simulink model "bike_model_2states_smithSteering"  (R2018b)
settings: Solver=VariableStepAuto  StartTime=0.0  StopTime=sim_time  FixedStep=Ts/10  MaxStep=Ts/10
values from neighbouring files (symbols this model uses):
  A_bike = [0 g/h_real ; 1 0]    [configuration.m]
  B_bike = [1 ; 0]    [configuration.m]
  b_compFilter = 1.095    [configuration.m]    (also in configuration_pidTuning.m)
  b_real = 1.095    [configuration.m]    (also in configuration_pidTuning.m)
  C1_bike = a_real/(b_real*h_real)    (= 0.392543973584)    [configuration.m]
  C2_bike = 1/(b_real*h_real)    (= 1.15454109878)    [configuration.m]
  C_ini = [C1_bike*input_velocity C2_bike*input_velocity^2]    [configuration.m]
  complementary = 0.985    [configuration.m]    (also in configuration_pidTuning.m)
  D = zeros(3,1)    [configuration_pidTuning.m]
  D_steering_position = 0.0    (= 0)    [configuration.m]
  Dead_Band = [0.055, -0.055, 0.005]    [configuration.m]    (also in configuration_pidTuning.m)
  delay = 0.045    [configuration.m]    (also in configuration_pidTuning.m)
  delay_tf_steering = 0    [configuration.m]
  den_tf_steering = [1 245.9 0]    [configuration.m]
  den_tf_steering_dis = [den_tf_steering_dis 0] - [0 den_tf_steering_dis]    [configuration.m]
  direct_control = 1    [configuration.m]    (also in configuration_pidTuning.m)
  f_filter_phidot = 20    [configuration.m]
  filter_model = 1    [configuration.m]    (also in configuration_pidTuning.m)
  forward_motor_dynamics = 0    [configuration.m]    (also in configuration_pidTuning.m)
  forward_speed_offset = 0    [configuration.m]
  g = 9.81    [configuration.m]    (also in configuration_pidTuning.m)
  I_direct = 0.000227125326188444    (= 0.000227125326188)    [configuration.m]    (also in configuration_pidTuning.m)
  I_lat = 0.000115580509653549    (= 0.000115580509654)    [configuration.m]    (also in configuration_pidTuning.m)
  I_steering_position = 1    [configuration.m]    (also in simulate_bike.m = 30)
  IMU_height_model = 0.45    [configuration.m]    (also in configuration_pidTuning.m)
  IMU_height_real = 0.45    [configuration.m]    (also in configuration_pidTuning.m)
  initial_states = [deg2rad(-2) deg2rad(0) deg2rad(0)]    [configuration.m]    (also in configuration_pidTuning.m)
  input_velocity = 4    [configuration.m]    (also in configuration_pidTuning.m = 3)
  lambda_compFilter = deg2rad(70)    [configuration.m]    (also in configuration_pidTuning.m)
  lambda_real = deg2rad(70)    [configuration.m]    (also in configuration_pidTuning.m)
  lat_control = 0    [configuration.m]    (also in configuration_pidTuning.m = 1)
  look_ahead = 0    [configuration.m]    (also in configuration_pidTuning.m)
  lqr_gains = zeros(length(velocity_lqr),1+size(A_bike,1))    [lqr_design.m]
  max_handlebar = 40*(pi/180)    (= 0.698131700798)    [configuration.m]    (also in configuration_pidTuning.m)
  max_roll = pi/2    (= 1.57079632679)    [configuration.m]    (also in configuration_pidTuning.m)
  max_steering_motor_acc = inf    [configuration.m]    (also in configuration_pidTuning.m)
  max_steering_motor_speed = 0.9    [configuration.m]    (also in configuration_pidTuning.m = 7.5)
  min_handlebar = -max_handlebar    (= -0.698131700798)    [configuration.m]    (also in configuration_pidTuning.m)
  min_roll = - max_roll    (= -1.57079632679)    [configuration.m]    (also in configuration_pidTuning.m)
  min_steering_motor_acc = -inf    [configuration.m]    (also in configuration_pidTuning.m)
  min_steering_motor_speed = -0.9    [configuration.m]    (also in configuration_pidTuning.m = -7.5)
  noise = 0    [configuration.m]    (also in configuration_pidTuning.m)
  noise_acc = 2.4869e-05    [configuration.m]    (also in configuration_pidTuning.m)
  noise_encoder = 1e-7    (= 1e-07)    [configuration.m]    (also in configuration_pidTuning.m)
  noise_gyro = 0.005    [configuration.m]    (also in configuration_pidTuning.m = 0.0022)
  noise_hall = 0.0031    [configuration.m]    (also in configuration_pidTuning.m)
  noise_pos_meas = 0    [configuration.m]    (also in configuration_pidTuning.m = 0.51)
  num_tf_steering = [253.4]    [configuration.m]
  num_tf_steering_dis = [num_tf_steering_dis 0]    [configuration.m]
  offset_acc = 0.0*g    (= 0)    [configuration.m]
  offset_encoder = deg2rad(1)    [configuration.m]
  offset_gyro = deg2rad(0)    [configuration.m]
  offset_hall = 0.0    (= 0)    [configuration.m]
  offset_pos_x = 0    [configuration.m]
  offset_pos_y = 0    [configuration.m]
  P_direct = 0.0712859744206787    (= 0.0712859744207)    [configuration.m]    (also in configuration_pidTuning.m)
  P_lat = 0.0465435246389258    (= 0.0465435246389)    [configuration.m]    (also in configuration_pidTuning.m)
  P_steering_position = 10    [configuration.m]    (also in simulate_bike.m = 30)
  parameters_compFilter = [g h_compFilter b_compFilter a_compFilter lambda_compFilter c_compFilter]    [configuration.m]    (also in configuration_pidTuning.m)
  roll_rate_coef = 0.9    [configuration.m]    (also in configuration_pidTuning.m)
  sensor_offset = 0    [configuration.m]
  smith_steering = 0    [configuration.m]
  steering_angle_correction = deg2rad(0)    [configuration.m]
  steering_motor_limitations = 0    [configuration.m]    (also in configuration_pidTuning.m = 1)
  sys_con = ss(A_lqr,B_lqr,C_lqr,D_lqr)    [lqr_design.m]
  time_offset_acc = 7    [configuration.m]
  time_offset_encoder = 10    [configuration.m]
  time_offset_gyro = 7    [configuration.m]
  time_offset_hall = 7    [configuration.m]
  time_offset_pos_x = 7    [configuration.m]
  time_offset_pos_y = 7    [configuration.m]
  Ts = 0.01    [configuration.m]    (also in configuration_pidTuning.m = 0.04)
  Ts_IMU = 0.01    [configuration.m]    (also in configuration_pidTuning.m = 0.04)
  velocity_lqr = [input_velocity - 0.1 , input_velocity , input_velocity + 0.1]    [lqr_design.m]
undefined symbols (not defined in the file or in its folder): A, B, cumulative_dist_along_path, curvature, den_filter_phidot, initial_x, initial_y, num_filter_phidot, path_x, path_y
libraries: simulink x17, simulink_extras x3, dspsigops x2
(part 2 of 3)

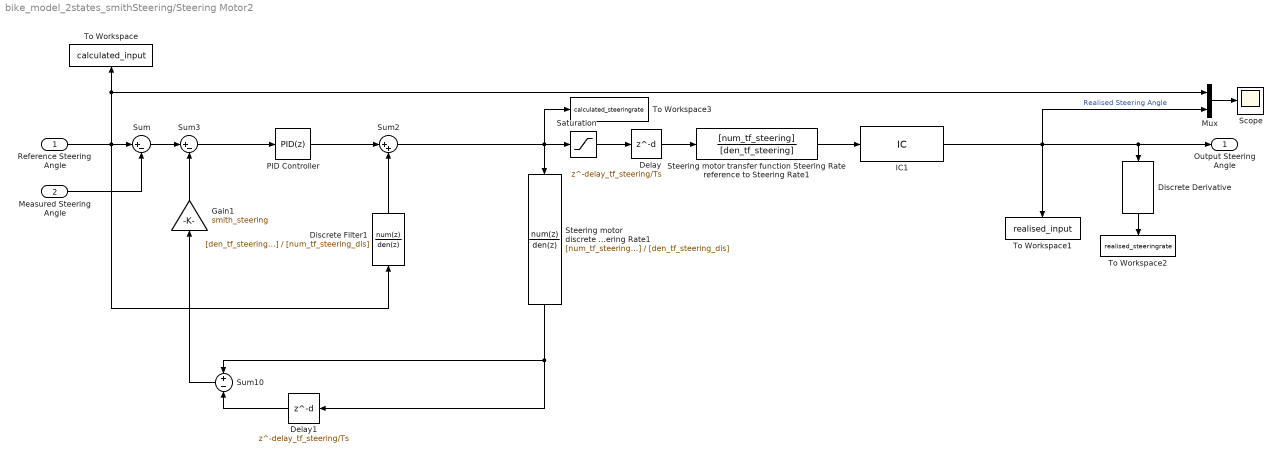
== system bike_model_2states_smithSteering/Steering Motor2 ==
  Reference Steering Angle : Inport
  Measured Steering Angle : Inport  Port=2
  Delay : Delay  DelayLength=delay_tf_steering/Ts  SampleTime=Ts
  Delay1 : Delay  DelayLength=delay_tf_steering/Ts  SampleTime=Ts
  Discrete Derivative : simulink/Discrete/Discrete Derivative  gainval=1.0  ICPrevScaledInput=0.0  OutMin=[]  OutMax=[]  OutDataType=fixdt(1, 16)  OutScaling=2^-10  DoSatur=off
  Discrete Filter1 : DiscreteFilter  Numerator=[den_tf_steering_dis]  Denominator=[num_tf_steering_dis]
  Gain1 : Gain  Gain=smith_steering
  IC1 : InitialCondition  Value=initial_states(2)
  Mux : Mux  Inputs=2
  PID Controller : simulink/Continuous/PID Controller  Controller=PID  Form=Parallel  TimeDomain=Discrete-time  SampleTime=Ts  IntegratorMethod=Forward Euler  FilterMethod=Forward Euler  ControllerParametersSource=internal  P=P_steering_position  I=I_steering_position  D=D_steering_position  UseFilter=off  N=1  TunerSelectOption=Transfer Function Based (PID Tuner App)  InitialConditionSource=internal  InitialConditionForIntegrator=0  InitialConditionForFilter=0  DifferentiatorICPrevScaledInput=0  ExternalReset=none  TrackingMode=off  Kt=1  LimitOutput=off  UpperSaturationLimit=inf  LowerSaturationLimit=-inf  LinearizeAsGain=on  AntiWindupMode=none  Kb=1  POutMin=[]  POutMax=[]  IOutMin=[]  IOutMax=[]  DOutMin=[]  DOutMax=[]  NOutMin=[]  NOutMax=[]  SumOutMin=[]  SumOutMax=[]  SaturationOutMin=[]  SaturationOutMax=[]  PParamMin=[]  PParamMax=[]  IParamMin=[]  IParamMax=[]  DParamMin=[]  DParamMax=[]  NParamMin=[]  NParamMax=[]  KbParamMin=[]  KbParamMax=[]  KtParamMin=[]  KtParamMax=[]  KbOutMin=[]  KbOutMax=[]  KtOutMin=[]  KtOutMax=[]  IntegratorOutMin=[]  IntegratorOutMax=[]  FilterOutMin=[]  FilterOutMax=[]  SumI1OutMin=[]  SumI1OutMax=[]  SumI2OutMin=[]  SumI2OutMax=[]  SumI3OutMin=[]  SumI3OutMax=[]  SumI4OutMin=[]  SumI4OutMax=[]  SumDOutMin=[]  SumDOutMax=[]  DifferentiatorOutMin=[]  DifferentiatorOutMax=[]  FilterDiffOutCoefMin=[]  FilterDiffOutCoefMax=[]  ReciprocalOutMin=[]  ReciprocalOutMax=[]  SumDenOutMin=[]  SumDenOutMax=[]  SumNumOutMin=[]  SumNumOutMax=[]  DivideOutMin=[]  DivideOutMax=[]  IntegratorContinuousStateAttributes=''  IntegratorStateMustResolveToSignalObject=off  IntegratorRTWStateStorageClass=Auto  FilterContinuousStateAttributes=''  FilterStateMustResolveToSignalObject=off  FilterRTWStateStorageClass=Auto  ParallelPVariant=InternalParameters  IdealPVariant=Disabled  IVariant=InternalParameters  DVariant=InternalParameters  IntegratorVariant=Discrete  SatVariant=Disabled  AWVariant=Passthrough  PCopyVariant=Disabled  TRVariant=Disabled  FdbkBlocksVariant=Forward  IdealPFdbkVariant=Disabled  SatFdbkVariant=Disabled  DerivativeFilterVariant=Differentiator  NVariant=Passthrough  NCopyVariant=Disabled_SignalSpec  FilterICVariant=InternalICsDifferentiator  IntegratorICVariant=InternalICs  ExternalResetVariant=Disabled  TRSumVariant=Passthrough  SumFdbkVariant=Disabled  SumVariant=Sum_PID
  Saturation : Saturate  UpperLimit=max_steering_motor_speed  LowerLimit=min_steering_motor_speed
  Scope : Scope
  Steering motor discrete transfer function Steering Rate reference to Steering Rate1 : DiscreteTransferFcn  Numerator=[num_tf_steering_dis]  Denominator=[den_tf_steering_dis]  SampleTime=Ts
  Steering motor transfer function Steering Rate reference to Steering Rate1 : TransferFcn  Numerator=[num_tf_steering]  Denominator=[den_tf_steering]
  Sum : Sum  Inputs=|+-
  Sum10 : Sum  Inputs=+-
  Sum2 : Sum  Inputs=|++
  Sum3 : Sum  Inputs=|+-
  To Workspace : ToWorkspace  VariableName=calculated_input  SaveFormat=Timeseries  SampleTime=Ts
  To Workspace1 : ToWorkspace  VariableName=realised_input  SaveFormat=Timeseries  SampleTime=-1
  To Workspace2 : ToWorkspace  VariableName=realised_steeringrate  SaveFormat=Timeseries  SampleTime=-1
  To Workspace3 : ToWorkspace  VariableName=calculated_steeringrate  SaveFormat=Timeseries  SampleTime=-1
  Output Steering Angle : Outport
  wires:
  Mux/1 -> Scope/1
  Delay/1 -> Steering motor transfer function Steering Rate reference to Steering Rate1/1
  PID Controller/1 -> Sum2/1
  Reference Steering Angle/1 -> Discrete Filter1/1, Sum/1, Mux/1, To Workspace/1
  Sum2/1 -> To Workspace3/1, Steering motor discrete transfer function Steering Rate reference to Steering Rate1/1, Saturation/1
  Measured Steering Angle/1 -> Sum/2
  Sum/1 -> Sum3/1
  Delay1/1 -> Sum10/2
  Steering motor discrete transfer function Steering Rate reference to Steering Rate1/1 -> Delay1/1, Sum10/1
  Sum10/1 -> Gain1/1
  Steering motor transfer function Steering Rate reference to Steering Rate1/1 -> IC1/1
  IC1/1 -> To Workspace1/1, Discrete Derivative/1, Output Steering Angle/1, Mux/2  "Realised Steering Angle"
  Discrete Filter1/1 -> Sum2/2
  Sum3/1 -> PID Controller/1
  Saturation/1 -> Delay/1
  Discrete Derivative/1 -> To Workspace2/1
  Gain1/1 -> Sum3/2

== system bike_model_2states_smithSteering/Balance Controller/LQR Controller ==
  note: Input = steering angular velocity
  Velocity : Inport
  State Error : Inport  Port=2
  1-D Lookup Table : Lookup_n-D  NumberOfTableDimensions=1  BreakpointsForDimension1=velocity_lqr  BreakpointsForDimension2=velocity_lqr  BreakpointsForDimension3=velocity_lqr  BreakpointsForDimension4=velocity_lqr  Table=lqr_gains(:,1)  InternalRulePriority=Speed  RndMeth=Simplest  InputSameDT=on
  1-D Lookup Table1 : Lookup_n-D  NumberOfTableDimensions=1  BreakpointsForDimension1=velocity_lqr  BreakpointsForDimension2=velocity_lqr  BreakpointsForDimension3=velocity_lqr  BreakpointsForDimension4=velocity_lqr  Table=lqr_gains(:,2)  InternalRulePriority=Speed  RndMeth=Simplest  InputSameDT=on
  Display1 : Display
  Mux : Mux  Inputs=2
  Product : Product  Multiplication=Matrix(*)
  Scope : Scope
  Transpose : Math  Operator=transpose  SaturateOnIntegerOverflow=on
  Zero-Order Hold : ZeroOrderHold  SampleTime=Ts
  Zero-Order Hold1 : ZeroOrderHold  SampleTime=Ts
  Calculated Input : Outport
  wires:
  1-D Lookup Table/1 -> Mux/1  "K1"
  1-D Lookup Table1/1 -> Mux/2  "K2"
  State Error/1 -> Zero-Order Hold1/1
  Product/1 -> Zero-Order Hold/1
  Velocity/1 -> 1-D Lookup Table1/1, 1-D Lookup Table/1
  Mux/1 -> Product/2, Display1/1
  Transpose/1 -> Product/1
  Zero-Order Hold/1 -> Calculated Input/1
  Zero-Order Hold1/1 -> Scope/1, Transpose/1

== system bike_model_2states_smithSteering/Balance Controller/Reference States Generator ==
  Velocity : Inport
  Steering Angle : Inport  Port=2
  Angles Error : Inport  Port=3
  Constant1 : Constant  Value=A_bike
  Constant2 : Constant  Value=0
  Constant3 : Constant  Value=B_bike
  Gain : Gain  Gain=C2_bike
  Gain1 : Gain  Gain=C1_bike
  Matrix Concatenate : Concatenate  Mode=Multidimensional array
  Mux1 : Mux  Inputs=2
  Mux2 : Mux  Inputs=2
  Product{1..4} (4 alike) : Product  SCDEnableBlockLinearizationSpecification=on  Multiplication=Matrix(*)
  Product5 : Product  SCDEnableBlockLinearizationSpecification=on  Inputs=/  Multiplication=Matrix(*)
  Reshape : Reshape  OutputDimensionality=Row vector (2-D)
  Square1 : Math  Operator=square  SaturateOnIntegerOverflow=on
  Sum : Sum  Inputs=-+
  State Error : Outport
  wires:
  Velocity/1 -> Square1/1, Gain1/1
  Square1/1 -> Gain/1
  Reshape/1 -> Product4/1, Matrix Concatenate/1, Product3/1  "C"
  Mux2/1 -> Reshape/1
  Constant1/1 -> Product3/2  "A"
  Product3/1 -> Matrix Concatenate/2  "CA"
  Matrix Concatenate/1 -> Product5/1  "[C ; CA]"
  Angles Error/1 -> Sum/2
  Product2/1 -> Sum/1
  Steering Angle/1 -> Product2/2
  Mux1/1 -> Product2/1  "[0 ; CB]"
  Constant2/1 -> Mux1/1
  Product4/1 -> Mux1/2
  Constant3/1 -> Product4/2  "B"
  Sum/1 -> Product1/2
  Product1/1 -> State Error/1  "CA"
  Product5/1 -> Product1/1  "CA"
  Gain1/1 -> Mux2/1
  Gain/1 -> Mux2/2

== system bike_model_2states_smithSteering/Balance Controller1/LQR Controller ==
  Velocity : Inport
  State Error : Inport  Port=2
  1-D Lookup Table : Lookup_n-D  NumberOfTableDimensions=1  BreakpointsForDimension1=velocity_lqr  BreakpointsForDimension2=velocity_lqr  BreakpointsForDimension3=velocity_lqr  BreakpointsForDimension4=velocity_lqr  Table=lqr_gains(:,2)  InternalRulePriority=Speed  RndMeth=Simplest  InputSameDT=on
  1-D Lookup Table1 : Lookup_n-D  NumberOfTableDimensions=1  BreakpointsForDimension1=velocity_lqr  BreakpointsForDimension2=velocity_lqr  BreakpointsForDimension3=velocity_lqr  BreakpointsForDimension4=velocity_lqr  Table=lqr_gains(:,3)  InternalRulePriority=Speed  RndMeth=Simplest  InputSameDT=on
  Display1 : Display
  Mux : Mux  Inputs=2
  Product : Product  Multiplication=Matrix(*)
  Transpose : Math  Operator=transpose  SaturateOnIntegerOverflow=on
  Zero-Order Hold : ZeroOrderHold  SampleTime=Ts
  Calculated Input : Outport
  wires:
  1-D Lookup Table/1 -> Mux/1  "K1"
  1-D Lookup Table1/1 -> Mux/2  "K2"
  Product/1 -> Zero-Order Hold/1
  Velocity/1 -> 1-D Lookup Table1/1, 1-D Lookup Table/1
  Mux/1 -> Product/2, Display1/1
  Transpose/1 -> Product/1
  Zero-Order Hold/1 -> Calculated Input/1
  State Error/1 -> Transpose/1

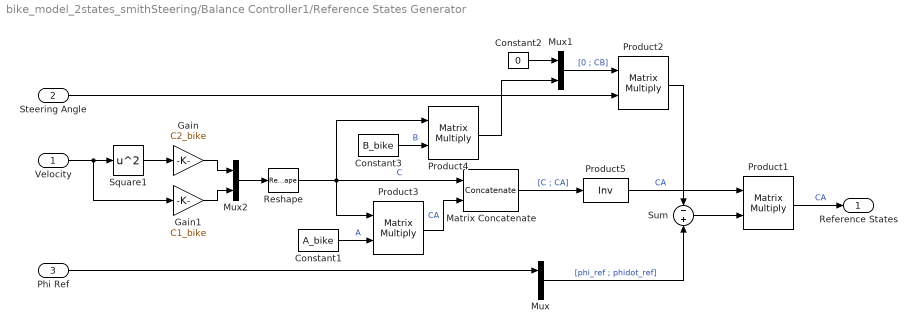
== system bike_model_2states_smithSteering/Balance Controller1/Reference States Generator ==
  Velocity : Inport
  Steering Angle : Inport  Port=2
  Phi Ref : Inport  Port=3
  Constant1 : Constant  Value=A_bike
  Constant2 : Constant  Value=0
  Constant3 : Constant  Value=B_bike
  Gain : Gain  Gain=C2_bike
  Gain1 : Gain  Gain=C1_bike
  Matrix Concatenate : Concatenate  Mode=Multidimensional array
  Mux : Mux  Inputs=2
  Mux1 : Mux  Inputs=2
  Mux2 : Mux  Inputs=2
  Product{1..4} (4 alike) : Product  SCDEnableBlockLinearizationSpecification=on  Multiplication=Matrix(*)
  Product5 : Product  SCDEnableBlockLinearizationSpecification=on  Inputs=/  Multiplication=Matrix(*)
  Reshape : Reshape  OutputDimensionality=Row vector (2-D)
  Square1 : Math  Operator=square  SaturateOnIntegerOverflow=on
  Sum : Sum  Inputs=-+
  Reference States : Outport
  wires:
  Velocity/1 -> Gain1/1, Square1/1
  Gain1/1 -> Mux2/2
  Gain/1 -> Mux2/1
  Square1/1 -> Gain/1
  Reshape/1 -> Product4/1, Matrix Concatenate/1, Product3/1  "C"
  Mux2/1 -> Reshape/1
  Constant1/1 -> Product3/2  "A"
  Product3/1 -> Matrix Concatenate/2  "CA"
  Matrix Concatenate/1 -> Product5/1  "[C ; CA]"
  Mux/1 -> Sum/2  "[phi_ref ; phidot_ref]"
  Phi Ref/1 -> Mux/1
  Product2/1 -> Sum/1
  Steering Angle/1 -> Product2/2
  Mux1/1 -> Product2/1  "[0 ; CB]"
  Constant2/1 -> Mux1/1
  Product4/1 -> Mux1/2
  Constant3/1 -> Product4/2  "B"
  Sum/1 -> Product1/2
  Product1/1 -> Reference States/1  "CA"
  Product5/1 -> Product1/1  "CA"

== system bike_model_2states_smithSteering/Complementary filter/Complementary Filter ==
  Roll Angle Estimation due to Accelerometer : Inport
  Roll Rate due to Gyroscope : Inport  Port=2
  Delay : Delay  DelayLength=1  InitialCondition=initial_states(1)
  Gain2 : Gain  Gain=complementary
  Gain3 : Gain  Gain=1-complementary
  Gain4 : Gain  Gain=Ts_IMU
  Sum3 : Sum  Inputs=|++
  Sum4 : Sum  Inputs=++|
  Roll Angle Estimation : Outport
  wires:
  Roll Angle Estimation due to Accelerometer/1 -> Gain3/1  "Roll_acc"
  Sum3/1 -> Gain2/1
  Roll Rate due to Gyroscope/1 -> Gain4/1
  Delay/1 -> Sum3/2
  Gain4/1 -> Sum3/1
  Gain2/1 -> Sum4/2
  Gain3/1 -> Sum4/1
  Sum4/1 -> Delay/1, Roll Angle Estimation/1

== system bike_model_2states_smithSteering/Complementary filter/Roll Angle Estimation of Accelerometer ==
  Accelerations : Inport
  Measured Steering Angle : Inport  Port=2
  Measured Velocity : Inport  Port=3
  Steering Rate : Inport  Port=4
  Roll Rate : Inport  Port=5
  Measured Roll Angle : Inport  Port=6
  Atan2 : Trigonometry  Operator=atan2
  Centripetal Acceleration Compensator : Subsystem
  Cos : Trigonometry  Operator=cos
  Demux : Demux  Outputs=3
  Lateral Acceleration Compensator : Subsystem
  Multiply : Product
  Multiply1 : Product
  Sin : Trigonometry
  Sum1 : Sum  Inputs=-+
  Sum6 : Sum  Inputs=+-+
  Roll Angle Estimation of Accelerometer : Outport
  wires:
  Sum1/1 -> Atan2/2
  Lateral Acceleration Compensator/1(Estimated Lateral Accelerattion due to Roll) -> Sum6/1
  Atan2/1 -> Roll Angle Estimation of Accelerometer/1  "Roll_acc"
  Roll Rate/1 -> Lateral Acceleration Compensator/4(Roll Rate)
  Accelerations/1 -> Demux/1
  Measured Velocity/1 -> Lateral Acceleration Compensator/1(Measured Velocity), Centripetal Acceleration Compensator/2(Velocity)
  Measured Steering Angle/1 -> Lateral Acceleration Compensator/3(Steering Angle), Centripetal Acceleration Compensator/1(Steering Angle)
  Centripetal Acceleration Compensator/1(Estimated Centripetal Acceleration) -> Multiply/2, Multiply1/1
  Measured Roll Angle/1 -> Lateral Acceleration Compensator/2(Roll Angle), Sin/1, Cos/1
  Cos/1 -> Multiply1/2
  Sin/1 -> Multiply/1
  Multiply1/1 -> Sum6/2
  Demux/3 -> Sum1/2
  Multiply/1 -> Sum1/1
  Steering Rate/1 -> Lateral Acceleration Compensator/5(Steering Rate)
  Sum6/1 -> Atan2/1
  Demux/2 -> Sum6/3

== system bike_model_2states_smithSteering/Complementary filter2/Complementary Filter ==
  Roll Angle Estimation due to Accelerometer : Inport
  Roll Rate due to Gyroscope : Inport  Port=2
  Delay : Delay  DelayLength=1  InitialCondition=initial_states(1)
  Gain2 : Gain  Gain=complementary
  Gain3 : Gain  Gain=1-complementary
  Gain4 : Gain  Gain=Ts_IMU
  Sum3 : Sum  Inputs=|++
  Sum4 : Sum  Inputs=++|
  Roll Angle Estimation : Outport
  wires:
  Roll Angle Estimation due to Accelerometer/1 -> Gain3/1  "Roll_acc"
  Sum3/1 -> Gain2/1
  Roll Rate due to Gyroscope/1 -> Gain4/1
  Delay/1 -> Sum3/2
  Gain4/1 -> Sum3/1
  Gain2/1 -> Sum4/2
  Gain3/1 -> Sum4/1
  Sum4/1 -> Delay/1, Roll Angle Estimation/1

== system bike_model_2states_smithSteering/Complementary filter2/Roll Angle Estimation of Accelerometer ==
  Accelerations : Inport
  Roll Rate : Inport  Port=2
  Measured Steering Angle : Inport  Port=3
  Measured Velocity : Inport  Port=4
  Measured Roll Angle : Inport  Port=5
  Steering Rate : Inport  Port=6
  Atan2 : Trigonometry  Operator=atan2
  Centripetal Acceleration Compensator : Subsystem
  Cos : Trigonometry  Operator=cos
  Demux : Demux  Outputs=3
  Lateral Acceleration Compensator : Subsystem
  Multiply : Product
  Multiply1 : Product
  Saturation -90°/90° : Saturate  UpperLimit=max_roll  LowerLimit=min_roll
  Sin : Trigonometry
  Sum1 : Sum  Inputs=-+
  Sum6 : Sum  Inputs=+-+
  Roll Angle Estimation of Accelerometer : Outport
  wires:
  Sum1/1 -> Atan2/2
  Lateral Acceleration Compensator/1(Estimated Lateral Accelerattion due to Roll) -> Sum6/1
  Atan2/1 -> Saturation -90°/90°/1  "Roll_acc"
  Roll Rate/1 -> Lateral Acceleration Compensator/4(Roll Rate)
  Accelerations/1 -> Demux/1
  Measured Velocity/1 -> Lateral Acceleration Compensator/1(Measured Velocity), Centripetal Acceleration Compensator/2(Velocity)
  Measured Steering Angle/1 -> Lateral Acceleration Compensator/3(Steering Angle)
  Centripetal Acceleration Compensator/1(Estimated Centripetal Acceleration) -> Multiply/2, Multiply1/1
  Measured Roll Angle/1 -> Lateral Acceleration Compensator/2(Roll Angle), Sin/1, Cos/1
  Cos/1 -> Multiply1/2
  Sin/1 -> Multiply/1
  Multiply1/1 -> Sum6/2
  Demux/3 -> Sum1/2
  Multiply/1 -> Sum1/1
  Steering Rate/1 -> Lateral Acceleration Compensator/5(Steering Rate)
  Sum6/1 -> Atan2/1
  Lateral Acceleration Compensator/2(Steering Angle (temporary output)) -> Centripetal Acceleration Compensator/1(Steering Angle)
  Demux/2 -> Sum6/3
  Saturation -90°/90°/1 -> Roll Angle Estimation of Accelerometer/1

== system bike_model_2states_smithSteering/Global Angles and Coordinates Calculator - Velocity/Measured Bike Angles to Global Angles ==
  note: Verification of the equivalence of the calculus for Beta estimation
  Velocity : Inport
  Measured Steering Angle : Inport  Port=2
  Gain : Gain  Gain=1/b_compFilter
  Integrator : Integrator
  MATLAB Function : MATLAB Function  TreatAsAtomicUnit=on
  Multiply : Product
  Parameters : Constant  Value=parameters_compFilter
  Scope : Scope  NumInputPorts=2
  Tan : Trigonometry  Operator=tan
  Psi : Outport
  Beta : Outport  Port=2
  wires:
  Integrator/1 -> Psi/1
  MATLAB Function/1(psi_d) -> Scope/1, Integrator/1
  Measured Steering Angle/1 -> Tan/1, MATLAB Function/3(delta)
  Parameters/1 -> MATLAB Function/2(parameters_model)
  Velocity/1 -> Multiply/1, MATLAB Function/1(v)
  MATLAB Function/2(beta) -> Beta/1
  Tan/1 -> Multiply/2
  Multiply/1 -> Gain/1
  Gain/1 -> Scope/2

== system bike_model_2states_smithSteering/Global Angles and Coordinates Calculator - Velocity/Measured Global Angles to Global Coordinates ==
  Velocity : Inport
  Psi : Inport  Port=2
  Beta : Inport  Port=3
  MATLAB Function1 : MATLAB Function  TreatAsAtomicUnit=on
  Mux1 : Mux  Inputs=2
  "Velocity (Xdot, Ydot)" : Outport
  wires:
  MATLAB Function1/2(Ydot) -> Mux1/2  "Ydot"
  MATLAB Function1/1(Xdot) -> Mux1/1  "Xdot"
  Psi/1 -> MATLAB Function1/2(psi)
  Beta/1 -> MATLAB Function1/3(beta)
  Velocity/1 -> MATLAB Function1/1(v)
  Mux1/1 -> "Velocity (Xdot, Ydot)"/1

== system bike_model_2states_smithSteering/IMU/IMU Accelerometer ==
  Lateral Acceleration of the IMU due to Roll : Inport
  Centripetal Acceleration due to Path Curvature : Inport  Port=2
  True Velocity : Inport  Port=3
  True Roll Angle : Inport  Port=4
  Cos : Trigonometry  Operator=cos
  Derivative : Derivative  CoefficientInTFapproximation=-1
  Gain1 : Gain  Gain=g
  Gain2 : Gain  Gain=g
  Multiply : Product
  Multiply1 : Product
  Mux : Mux  Inputs=3
  Sin : Trigonometry
  Sum1 : Sum  Inputs=-+
  Sum6 : Sum  Inputs=-++
  Accelerations : Outport
  wires:
  Multiply/1 -> Sum6/2
  Gain1/1 -> Sum6/3  "acc_y"
  Sin/1 -> Multiply1/2, Gain1/1
  Derivative/1 -> Mux/1  "acc_x"
  Cos/1 -> Multiply/2, Gain2/1
  Gain2/1 -> Sum1/2  "acc_z"
  True Roll Angle/1 -> Sin/1, Cos/1
  True Velocity/1 -> Derivative/1
  Centripetal Acceleration due to Path Curvature/1 -> Multiply1/1, Multiply/1
  Multiply1/1 -> Sum1/1
  Sum1/1 -> Mux/3
  Mux/1 -> Accelerations/1
  Sum6/1 -> Mux/2
  Lateral Acceleration of the IMU due to Roll/1 -> Sum6/1

== system bike_model_2states_smithSteering/IMU/IMU Gyroscope ==
  True Velocity : Inport
  True Roll Angle : Inport  Port=2
  True Roll Rate : Inport  Port=3
  Measured Steering Angle : Inport  Port=4
  "Bike Model b " : Constant  Value=b_compFilter
  Cos : Trigonometry  Operator=cos
  Divide : Product  Inputs=*/
  Gain : Gain  Gain=sin(lambda_compFilter)
  Low-pass Filter : TransferFcn  Numerator=num_filter_phidot  Denominator=den_filter_phidot
  Multiply : Product
  Multiply1 : Product
  Multiply2 : Product
  Mux : Mux  Inputs=3
  Sin : Trigonometry
  Tan : Trigonometry  Operator=tan
  Transfer Fcn : TransferFcn  Denominator=[1/(2*pi*f_filter_phidot) 1]
  Angular rates : Outport
  wires:
  Mux/1 -> Angular rates/1
  Tan/1 -> Multiply/1
  Gain/1 -> Tan/1
  Measured Steering Angle/1 -> Gain/1
  Cos/1 -> Multiply1/1
  True Roll Angle/1 -> Sin/1, Cos/1
  Sin/1 -> Multiply2/1
  True Velocity/1 -> Divide/1
  "Bike Model b "/1 -> Divide/2
  Divide/1 -> Multiply/2  "v/b"
  Multiply/1 -> Multiply2/2, Multiply1/2
  Multiply2/1 -> Mux/2
  Multiply1/1 -> Mux/3
  True Roll Rate/1 -> Mux/1, Transfer Fcn/1, Low-pass Filter/1

== system bike_model_2states_smithSteering/Path Tracking Controller1/Lateral Error ==
  Psi Sigma : Inport
  Position Error (X,Y) : Inport  Port=2
  Cos : Trigonometry  Operator=cos
  Demux : Demux  Outputs=2
  Product : Product
  Product1 : Product
  Sin : Trigonometry
  Sum : Sum  Inputs=+-|
  To Workspace4 : ToWorkspace  VariableName=LAT_ERR  SaveFormat=Timeseries  SampleTime=Ts
  Lateral Error : Outport
  wires:
  Cos/1 -> Product/2
  Sin/1 -> Product1/1
  Psi Sigma/1 -> Cos/1, Sin/1
  Product1/1 -> Sum/2
  Product/1 -> Sum/1
  Sum/1 -> To Workspace4/1, Lateral Error/1  "Lateral Error"
  Demux/1 -> Product1/2  "X Position Error"
  Demux/2 -> Product/1  "Y Position Error"
  Position Error (X,Y)/1 -> Demux/1

== system bike_model_2states_smithSteering/Physical Bike/Centripetal Acceleration Calculator ==
  True Steering Angle : Inport
  True Velocity : Inport  Port=2
  Divide : Product  Inputs=*/
  Gain : Gain  Gain=sin(lambda_real)
  Multiply : Product
  Square : Math  Operator=square  SaturateOnIntegerOverflow=on
  Tan : Trigonometry  Operator=tan
  b Real Bike : Constant  Value=b_real
  Centripetal Acceleration : Outport
  wires:
  True Velocity/1 -> Square/1
  Square/1 -> Divide/1
  b Real Bike/1 -> Divide/2
  True Steering Angle/1 -> Gain/1
  Divide/1 -> Multiply/1
  Tan/1 -> Multiply/2
  Multiply/1 -> Centripetal Acceleration/1
  Gain/1 -> Tan/1

== system bike_model_2states_smithSteering/Physical Bike/Check Phi Limits ==
  x : Inport
  Roll Lower Bound : simulink/Model Verification/Check Static  Lower Bound  Description=min_roll <= u  min=min_roll  min_included=on  enabled=on  stopWhenAssertionFail=on  export=off  icon=graphic
      settings: SourceProductName=Simulink
  Roll Upper Bound : simulink/Model Verification/Check Static  Upper Bound  Description=u <= max_roll  max=max_roll  max_included=on  enabled=on  stopWhenAssertionFail=on  export=off  icon=graphic
      settings: SourceProductName=Simulink  SourceProductBaseCode=SL
  wires:
  x/1 -> Roll Lower Bound/1, Roll Upper Bound/1  "Roll Angle"

== system bike_model_2states_smithSteering/Physical Bike/Global Angles and Coordinates Calculator - Position ==
  note: True Steering
      | Angle
  True Velocity : Inport
  True Steering Angle : Inport  Port=2
  Gain1 : Gain  Gain=sin(lambda_compFilter)
  Measured Bike Angles to Global Angles : Subsystem
  Measured Global Angles to Global Coordinates : Subsystem
  Sum : Sum  Inputs=++|
  True Position : Outport
  True Heading : Outport  Port=2
  wires:
  Measured Bike Angles to Global Angles/1(Psi) -> Sum/2, Measured Global Angles to Global Coordinates/2(Psi)
  Gain1/1 -> Measured Bike Angles to Global Angles/2(Measured Steering Angle)
  Sum/1 -> True Heading/1
  Measured Bike Angles to Global Angles/2(Beta) -> Sum/1, Measured Global Angles to Global Coordinates/3(Beta)
  Measured Global Angles to Global Coordinates/1("Position (X, Y)") -> True Position/1
  True Velocity/1 -> Measured Global Angles to Global Coordinates/1(Velocity), Measured Bike Angles to Global Angles/1(Velocity)
  True Steering Angle/1 -> Gain1/1

== system bike_model_2states_smithSteering/Physical Bike/Lateral Acceleration (due to Roll) Calculator ==
  Roll Acceleration : Inport
  Constant3 : Constant  Value=IMU_height_real
  Multiply : Product
  Lateral Acceleration : Outport
  wires:
  Multiply/1 -> Lateral Acceleration/1
  Constant3/1 -> Multiply/1
  Roll Acceleration/1 -> Multiply/2

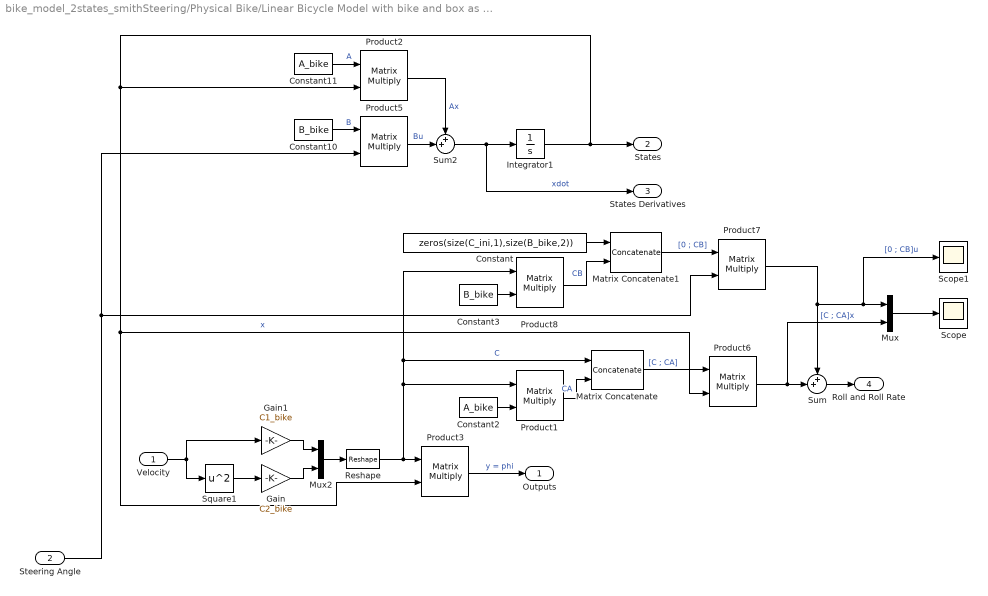
== system bike_model_2states_smithSteering/Physical Bike/Linear Bicycle Model with bike and box as 1 volume ==
  Velocity : Inport
  Steering Angle : Inport  Port=2
  Constant : Constant  Value=zeros(size(C_ini,1),size(B_bike,2))
  Constant10 : Constant  Value=B_bike
  Constant11 : Constant  Value=A_bike
  Constant2 : Constant  Value=A_bike
  Constant3 : Constant  Value=B_bike
  Gain : Gain  Gain=C2_bike
  Gain1 : Gain  Gain=C1_bike
  Integrator1 : Integrator  InitialCondition=[C_ini ; C_ini*A_bike]\[initial_states(1) ; initial_states(3)]
  Matrix Concatenate : Concatenate  Mode=Multidimensional array
  Matrix Concatenate1 : Concatenate  Mode=Multidimensional array
  Mux : Mux  Inputs=2
  Mux2 : Mux  Inputs=2
  Product{1..3,5..8} (7 alike) : Product  SCDEnableBlockLinearizationSpecification=on  Multiplication=Matrix(*)
  Reshape : Reshape  OutputDimensionality=Row vector (2-D)
  Scope : Scope
  Scope1 : Scope
  Square1 : Math  Operator=square  SaturateOnIntegerOverflow=on
  Sum : Sum  Inputs=++|
  Sum2 : Sum  Inputs=++|
  Outputs : Outport
  States : Outport  Port=2
  States Derivatives : Outport  Port=3
  Roll and Roll Rate : Outport  Port=4
  wires:
  Integrator1/1 -> Product2/2, Product6/2, Product3/2, States/1  "x"
  Product3/1 -> Outputs/1  "y = phi"
  Steering Angle/1 -> Product5/2, Product7/2
  Product2/1 -> Sum2/1  "Ax"
  Mux2/1 -> Reshape/1
  Product5/1 -> Sum2/2  "Bu"
  Sum2/1 -> Integrator1/1, States Derivatives/1  "xdot"
  Constant11/1 -> Product2/1  "A"
  Constant10/1 -> Product5/1  "B"
  Velocity/1 -> Gain1/1, Square1/1
  Square1/1 -> Gain/1
  Reshape/1 -> Product3/1, Product8/1, Matrix Concatenate/1, Product1/1  "C"
  Gain/1 -> Mux2/2
  Gain1/1 -> Mux2/1
  Sum/1 -> Roll and Roll Rate/1
  Constant2/1 -> Product1/2
  Product1/1 -> Matrix Concatenate/2  "CA"
  Matrix Concatenate/1 -> Product6/1  "[C ; CA]"
  Product6/1 -> Mux/2, Sum/2  "[C ; CA]x"
  Product7/1 -> Scope1/1, Mux/1, Sum/1  "[0 ; CB]u"
  Matrix Concatenate1/1 -> Product7/1  "[0 ; CB]"
  Product8/1 -> Matrix Concatenate1/2  "CB"
  Constant3/1 -> Product8/2
  Constant/1 -> Matrix Concatenate1/1
  Mux/1 -> Scope/1

== system bike_model_2states_smithSteering/Physical Bike/Path Plotter Reality ==
  Position : Inport
  Demux : Demux  Outputs=2
  To Workspace : ToWorkspace  VariableName=X_BIKE  SaveFormat=Timeseries  SampleTime=-1
  To Workspace1 : ToWorkspace  VariableName=Y_BIKE  SaveFormat=Timeseries  SampleTime=-1
  XY Graph : simulink/Sinks/XY Graph  Commented=on  xmin=min(path_x)-5  xmax=max(path_x)+5  ymin=min(path_y)-5  ymax=max(path_y)+5  st=-1
  wires:
  Demux/1 -> XY Graph/1, To Workspace/1  "X"
  Demux/2 -> XY Graph/2, To Workspace1/1  "Y"
  Position/1 -> Demux/1

== system bike_model_2states_smithSteering/Reference Position /Reference Position and Angle Selector ==
  total travelled distance : Inport
  1-D Lookup Table : Lookup_n-D  NumberOfTableDimensions=1  BreakpointsForDimension1=cumulative_dist_along_path  Table=path_x  ExtrapMethod=Clip  DiagnosticForOutOfRangeInput=Error  InternalRulePriority=Speed  RndMeth=Simplest  InputSameDT=on
  1-D Lookup Table1 : Lookup_n-D  NumberOfTableDimensions=1  BreakpointsForDimension1=cumulative_dist_along_path  Table=path_y  ExtrapMethod=Clip  DiagnosticForOutOfRangeInput=Error  InternalRulePriority=Speed  RndMeth=Simplest  InputSameDT=on
  Atan2 : Trigonometry  Operator=atan2
  Derivative : Derivative
  Derivative1 : Derivative
  Scope : Scope
  Unwrap : dspsigops/Unwrap  tol=pi  InputProcessing=Columns as channels (frame based)  running=off
  X_sigma : Outport
  Y_sigma : Outport  Port=2
  psi_sigma : Outport  Port=3
  wires:
  total travelled distance/1 -> 1-D Lookup Table1/1, 1-D Lookup Table/1
  Unwrap/1 -> Scope/1, psi_sigma/1
  1-D Lookup Table/1 -> X_sigma/1, Derivative1/1  "interpolated path x value"
  Derivative1/1 -> Atan2/2  "dx"
  Derivative/1 -> Atan2/1  "dy"
  Atan2/1 -> Unwrap/1
  1-D Lookup Table1/1 -> Y_sigma/1, Derivative/1  "interpolated path y value"

== system bike_model_2states_smithSteering/Reference Position /Subsystem1 ==
  total travelled distance : Inport
  1-D Lookup Table : Lookup_n-D  NumberOfTableDimensions=1  BreakpointsForDimension1=cumulative_dist_along_path  Table=path_x  ExtrapMethod=Clip  DiagnosticForOutOfRangeInput=Error  InternalRulePriority=Speed  RndMeth=Simplest  InputSameDT=on
  1-D Lookup Table1 : Lookup_n-D  NumberOfTableDimensions=1  BreakpointsForDimension1=cumulative_dist_along_path  Table=path_y  ExtrapMethod=Clip  DiagnosticForOutOfRangeInput=Error  InternalRulePriority=Speed  RndMeth=Simplest  InputSameDT=on
  Atan2 : Trigonometry  Operator=atan2
  Derivative : Derivative
  Derivative1 : Derivative
  Scope : Scope
  Unwrap : dspsigops/Unwrap  tol=pi  InputProcessing=Columns as channels (frame based)  running=off
  X_sigma : Outport
  Y_sigma : Outport  Port=2
  psi_sigma : Outport  Port=3
  wires:
  total travelled distance/1 -> 1-D Lookup Table1/1, 1-D Lookup Table/1
  Unwrap/1 -> Scope/1, psi_sigma/1
  1-D Lookup Table/1 -> X_sigma/1, Derivative1/1  "interpolated path x value"
  Derivative1/1 -> Atan2/2  "dx"
  Derivative/1 -> Atan2/1  "dy"
  Atan2/1 -> Unwrap/1
  1-D Lookup Table1/1 -> Y_sigma/1, Derivative/1  "interpolated path y value"

== system bike_model_2states_smithSteering/Reference Position /Variable Look Ahead ==
  Velocity : Inport
  Total Tavelled Distance : Inport  Port=2
  1-D Lookup Table2 : Lookup_n-D  NumberOfTableDimensions=1  BreakpointsForDimension1=cumulative_dist_along_path  Table=curvature  ExtrapMethod=Clip  DiagnosticForOutOfRangeInput=Error  InternalRulePriority=Speed  RndMeth=Simplest  InputSameDT=on
  Add1 : Sum
  Clock : Clock
  Delay : Delay  DelayLength=1
  Delay1 : Delay  DelayLength=1
  Demux3 : Demux  Outputs=2
  Gain : Gain  Gain=8
  Look Ahead Time for Curvature Check : Gain  Gain=3
  Look-Ahead Coefficient Selector : MATLAB Function  TreatAsAtomicUnit=on
  "Look-Ahead Coefficient Modifier (Slow Turn-Off) " : MATLAB Function  TreatAsAtomicUnit=on
  Mux1 : Mux  Inputs=2
  Product3 : Product
  Scope2 : Scope
  Look Ahead Distance : Outport
  wires:
  Look Ahead Time for Curvature Check/1 -> Add1/1
  Delay/1 -> "Look-Ahead Coefficient Modifier (Slow Turn-Off) "/2(feedback)
  "Look-Ahead Coefficient Modifier (Slow Turn-Off) "/1(look_ahead_modified) -> Delay/1, Gain/1
  Demux3/1 -> Look-Ahead Coefficient Selector/1(curv_next)
  Look-Ahead Coefficient Selector/1(look_ahead) -> "Look-Ahead Coefficient Modifier (Slow Turn-Off) "/1(look_ahead), Scope2/1
  Clock/1 -> "Look-Ahead Coefficient Modifier (Slow Turn-Off) "/3(time), Delay1/1
  Delay1/1 -> "Look-Ahead Coefficient Modifier (Slow Turn-Off) "/4(time_delayed)
  1-D Lookup Table2/1 -> Demux3/1
  Total Tavelled Distance/1 -> Add1/2, Mux1/2
  Demux3/2 -> Look-Ahead Coefficient Selector/2(curv)
  Gain/1 -> Product3/1  "Look-Ahead Time"
  Add1/1 -> Mux1/1
  Mux1/1 -> 1-D Lookup Table2/1
  Velocity/1 -> Product3/2, Look Ahead Time for Curvature Check/1
  Product3/1 -> Look Ahead Distance/1

== system bike_model_2states_smithSteering/Steering Motor1/Motor Deadband ==
  Calculated Input : Inport
  Abs : Abs
  Abs1 : Abs
  Constant : Constant  Value=0  SampleTime=Ts
  Constant1 : Constant  Value=0  SampleTime=Ts
  Constant2 : Constant  Value=Dead_Band(2)  SampleTime=Ts
  Constant4 : Constant  Value=Dead_Band(1)  SampleTime=Ts
  Gain : Gain  Gain=-1
  Relay1 : Relay  OnSwitchValue=Dead_Band(3)  OffSwitchValue=-Dead_Band(3)
  Relay2 : Relay  OnSwitchValue=Dead_Band(3)  OffSwitchValue=-Dead_Band(3)
  Sum1 : Sum  Inputs=-+|
  Sum2 : Sum  Inputs=-+|
  Switch : Switch  Criteria=u2 > Threshold
  Switch1 : Switch  Criteria=u2 > Threshold
  Switch2 : Switch  Criteria=u2 > Threshold
  Input Signal After Dead Band : Outport
  wires:
  Constant4/1 -> Sum1/1
  Sum1/1 -> Relay1/1
  Relay1/1 -> Switch/2
  Switch/1 -> Switch1/1
  Constant/1 -> Switch/3
  Switch1/1 -> Input Signal After Dead Band/1
  Switch2/1 -> Switch1/3
  Constant1/1 -> Switch2/3
  Gain/1 -> Sum2/1
  Calculated Input/1 -> Abs/1, Switch2/1, Abs1/1, Switch/1, Switch1/2
  Sum2/1 -> Relay2/1
  Relay2/1 -> Switch2/2
  Abs/1 -> Sum2/2
  Abs1/1 -> Sum1/2
  Constant2/1 -> Gain/1

== system bike_model_2states_smithSteering/Steering Motor1/Velocity Saturation wrt Max and Min Handle Bar Angles ==
  Reference Steering Rate : Inport
  States : Inport  Port=2
  AND : Logic  IconShape=distinctive  AllPortsSameDT=off  OutDataTypeStr=boolean
  AND1 : Logic  IconShape=distinctive  AllPortsSameDT=off  OutDataTypeStr=boolean
  Compare To Constant : simulink/Logic and Bit Operations/Compare To Constant  relop=>=  const=max_handlebar  OutDataTypeStr=boolean
  Compare To Constant1 : simulink/Logic and Bit Operations/Compare To Constant  relop=<=  const=min_handlebar  OutDataTypeStr=boolean
  Compare To Zero : simulink/Logic and Bit Operations/Compare To Zero  relop=>=  OutDataTypeStr=boolean
  Compare To Zero1 : simulink/Logic and Bit Operations/Compare To Zero  relop=<=  OutDataTypeStr=boolean
  Constant : Constant  Value=0
  Demux : Demux  Outputs=3
  OR : Logic  Operator=OR  IconShape=distinctive  AllPortsSameDT=off  OutDataTypeStr=boolean
  Switch : Switch  Criteria=u2 > Threshold
  Output Steering Rate : Outport
  wires:
  Switch/1 -> Output Steering Rate/1
  Constant/1 -> Switch/1
  States/1 -> Demux/1
  Compare To Constant/1 -> AND/2
  OR/1 -> Switch/2
  Reference Steering Rate/1 -> Switch/3, Compare To Zero/1, Compare To Zero1/1
  Compare To Constant1/1 -> AND1/1
  AND1/1 -> OR/2
  Demux/2 -> Compare To Constant/1, Compare To Constant1/1
  AND/1 -> OR/1
  Compare To Zero1/1 -> AND1/2
  Compare To Zero/1 -> AND/1

== system bike_model_2states_smithSteering/Complementary filter/Roll Angle Estimation of Accelerometer/Centripetal Acceleration Compensator ==
  Steering Angle : Inport
  Velocity : Inport  Port=2
  Bike Model b : Constant  Value=b_compFilter
  Divide : Product  Inputs=*/
  Gain : Gain  Gain=sin(lambda_compFilter)
  Multiply : Product
  Square : Math  Operator=square  SaturateOnIntegerOverflow=on
  Tan : Trigonometry  Operator=tan
  Estimated Centripetal Acceleration : Outport
  wires:
  Velocity/1 -> Square/1
  Square/1 -> Divide/1
  Bike Model b/1 -> Divide/2
  Steering Angle/1 -> Gain/1
  Divide/1 -> Multiply/1
  Tan/1 -> Multiply/2
  Multiply/1 -> Estimated Centripetal Acceleration/1
  Gain/1 -> Tan/1

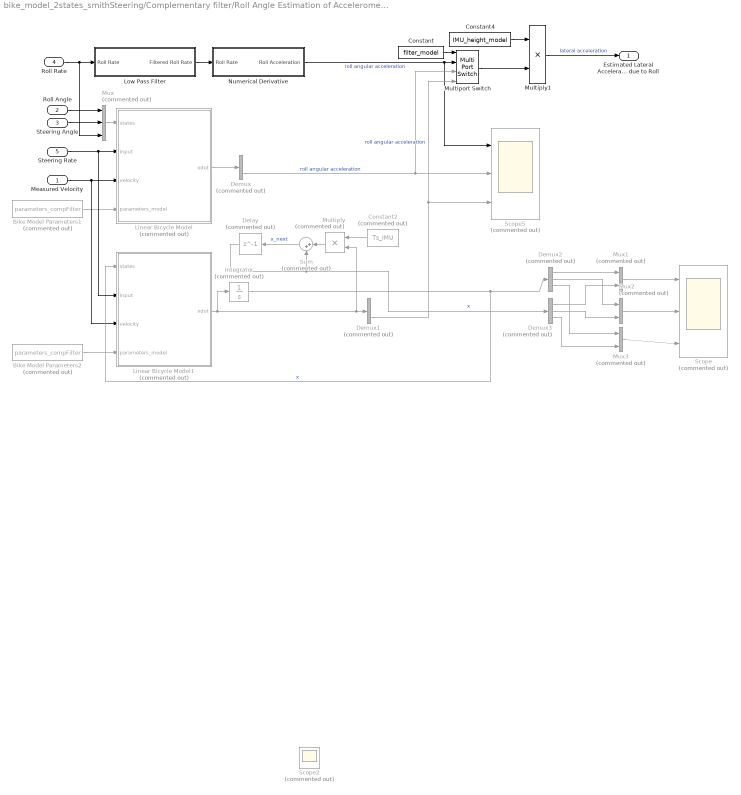
== system bike_model_2states_smithSteering/Complementary filter/Roll Angle Estimation of Accelerometer/Lateral Acceleration Compensator ==
  Measured Velocity : Inport
  Roll Angle : Inport  Port=2
  Steering Angle : Inport  Port=3
  Roll Rate : Inport  Port=4
  Steering Rate : Inport  Port=5
  Bike Model Parameters1 : Constant  Commented=on  Value=parameters_compFilter
  Bike Model Parameters2 : Constant  Commented=on  Value=parameters_compFilter
  Constant : Constant  Value=filter_model
  Constant2 : Constant  Commented=on  Value=Ts_IMU  SampleTime=Ts_IMU
  Constant4 : Constant  Value=IMU_height_model
  Delay : Delay  Commented=on  DelayLength=1  InitialCondition=[0 0 0]  SampleTime=Ts_IMU
  Demux{,1..3} (4 alike) : Demux  Commented=on  Outputs=3
  Integrator : Integrator  Commented=on  InitialCondition=initial_states
  Linear Bicycle Model : MATLAB Function  Commented=on  TreatAsAtomicUnit=on
  Linear Bicycle Model1 : MATLAB Function  Commented=on  TreatAsAtomicUnit=on
  Low Pass Filter : Subsystem
  Multiply : Product  Commented=on
  Multiply1 : Product
  Multiport Switch : MultiPortSwitch
  Mux : Mux  Commented=on  Inputs=3
  Mux1 : Mux  Commented=on  Inputs=2
  Mux2 : Mux  Commented=on  Inputs=2
  Mux3 : Mux  Commented=on  Inputs=2
  Numerical Derivative : Subsystem
  Scope : Scope  Commented=on  NumInputPorts=3
  Scope2 : Scope  Commented=on
  Scope5 : Scope  Commented=on  NumInputPorts=3
  Sum : Sum  Commented=on  Inputs=|++
  Estimated Lateral Accelerattion due to Roll : Outport
  wires:
  Numerical Derivative/1(Roll Acceleration) -> Scope5/1, Multiport Switch/2  "roll angular acceleration"
  Roll Rate/1 -> Mux/3, Low Pass Filter/1(Roll Rate)
  Constant4/1 -> Multiply1/1
  Multiply1/1 -> Estimated Lateral Accelerattion due to Roll/1  "lateral acceleration"
  Low Pass Filter/1(Filtered Roll Rate) -> Numerical Derivative/1(Roll Rate)
  Linear Bicycle Model/1(xdot) -> Demux/1
  Demux/3 -> Scope5/2, Multiport Switch/3  "roll angular acceleration"
  Bike Model Parameters1/1 -> Linear Bicycle Model/4(parameters_model)
  Measured Velocity/1 -> Linear Bicycle Model1/3(velocity), Linear Bicycle Model/3(velocity)
  Mux/1 -> Linear Bicycle Model/1(states)
  Roll Angle/1 -> Mux/1
  Steering Angle/1 -> Mux/2
  Constant/1 -> Multiport Switch/1
  Multiport Switch/1 -> Multiply1/2
  Demux1/3 -> Multiport Switch/4, Scope5/3  "roll angular acceleration"
  Bike Model Parameters2/1 -> Linear Bicycle Model1/4(parameters_model)
  Delay/1 -> Demux3/1, Sum/2  "x"
  Multiply/1 -> Sum/1
  Constant2/1 -> Multiply/1
  Integrator/1 -> Linear Bicycle Model1/1(states), Demux2/1  "x"
  Demux2/1 -> Mux1/1
  Demux3/1 -> Mux1/2
  Demux2/2 -> Mux2/1
  Demux3/2 -> Mux2/2
  Demux2/3 -> Mux3/1
  Demux3/3 -> Mux3/2
  Mux2/1 -> Scope/2
  Mux3/1 -> Scope/3
  Linear Bicycle Model1/1(xdot) -> Multiply/2, Demux1/1, Integrator/1
  Sum/1 -> Delay/1  "x_next"
  Steering Rate/1 -> Linear Bicycle Model1/2(input), Linear Bicycle Model/2(input)
  Mux1/1 -> Scope/1

== system bike_model_2states_smithSteering/Complementary filter2/Roll Angle Estimation of Accelerometer/Centripetal Acceleration Compensator ==
  Steering Angle : Inport
  Velocity : Inport  Port=2
  Bike Model b : Constant  Value=b_compFilter
  Divide : Product  Inputs=*/
  Gain : Gain  Gain=sin(lambda_compFilter)
  Multiply : Product
  Square : Math  Operator=square  SaturateOnIntegerOverflow=on
  Tan : Trigonometry  Operator=tan
  Estimated Centripetal Acceleration : Outport
  wires:
  Velocity/1 -> Square/1
  Square/1 -> Divide/1
  Bike Model b/1 -> Divide/2
  Steering Angle/1 -> Gain/1
  Divide/1 -> Multiply/1
  Tan/1 -> Multiply/2
  Multiply/1 -> Estimated Centripetal Acceleration/1
  Gain/1 -> Tan/1

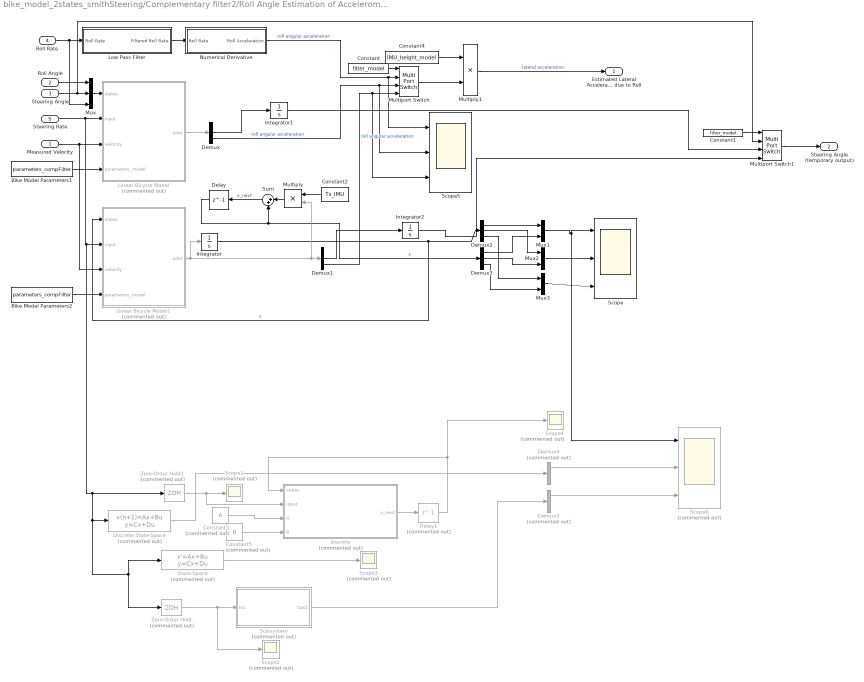
== system bike_model_2states_smithSteering/Complementary filter2/Roll Angle Estimation of Accelerometer/Lateral Acceleration Compensator ==
  Measured Velocity : Inport
  Roll Angle : Inport  Port=2
  Steering Angle : Inport  Port=3
  Roll Rate : Inport  Port=4
  Steering Rate : Inport  Port=5
  Bike Model Parameters1 : Constant  Value=parameters_compFilter
  Bike Model Parameters2 : Constant  Value=parameters_compFilter
  Constant : Constant  Value=filter_model
  Constant1 : Constant  Value=filter_model
  Constant2 : Constant  Value=Ts_IMU  SampleTime=Ts_IMU
  Constant3 : Constant  Commented=on  Value=A
  Constant4 : Constant  Value=IMU_height_model
  Constant5 : Constant  Commented=on  Value=B
  Delay : Delay  DelayLength=1  InitialCondition=[0 0 0]  SampleTime=Ts_IMU
  Delay1 : Delay  Commented=on  DelayLength=1  InitialCondition=[0 0 0]  SampleTime=Ts_IMU
  Demux{,1..3} (4 alike) : Demux  Outputs=3
  Demux4 : Demux  Commented=on  Outputs=3
  Demux5 : Demux  Commented=on  Outputs=3
  Discrete State-Space : DiscreteStateSpace  Commented=on  A=A  B=B  C=eye(3,3)  D=zeros(3,1)  InitialCondition=[0 0 0]  SampleTime=Ts_IMU
  Integrator : Integrator  InitialCondition=initial_states
  Integrator1 : Integrator  InitialCondition=initial_states(2)
  Integrator2 : Integrator  InitialCondition=initial_states(2)
  Linear Bicycle Model : MATLAB Function  Commented=on  TreatAsAtomicUnit=on
  Linear Bicycle Model1 : MATLAB Function  Commented=on  TreatAsAtomicUnit=on
  Low Pass Filter : Subsystem
  Multiply : Product
  Multiply1 : Product
  Multiport Switch : MultiPortSwitch
  Multiport Switch1 : MultiPortSwitch
  Mux : Mux  Inputs=3
  Mux1 : Mux  Inputs=2
  Mux2 : Mux  Inputs=2
  Mux3 : Mux  Inputs=2
  Numerical Derivative : Subsystem
  Scope : Scope  NumInputPorts=3
  Scope{1..4} (4 alike) : Scope  Commented=on
  Scope5 : Scope  NumInputPorts=3
  Scope6 : Scope  Commented=on  NumInputPorts=3
  State-Space : StateSpace  Commented=on  A=sys_con.A  B=sys_con.B  C=eye(3,3)  D=zeros(3,1)  InitialCondition=[0 0 0]
  Subsystem : Subsystem  Commented=on  TreatAsAtomicUnit=on  SystemSampleTime=Ts_IMU
  Sum : Sum  Inputs=|++
  Zero-Order Hold : ZeroOrderHold  Commented=on  SampleTime=Ts_IMU
  Zero-Order Hold1 : ZeroOrderHold  Commented=on  SampleTime=Ts_IMU
  discrete : MATLAB Function  Commented=on  TreatAsAtomicUnit=on
  Estimated Lateral Accelerattion due to Roll : Outport
  Steering Angle (temporary output) : Outport  Port=2
  wires:
  Numerical Derivative/1(Roll Acceleration) -> Scope5/1, Multiport Switch/2  "roll angular acceleration"
  Roll Rate/1 -> Mux/3, Low Pass Filter/1(Roll Rate)
  Constant4/1 -> Multiply1/1
  Multiply1/1 -> Estimated Lateral Accelerattion due to Roll/1  "lateral acceleration"
  Low Pass Filter/1(Filtered Roll Rate) -> Numerical Derivative/1(Roll Rate)
  Linear Bicycle Model/1(xdot) -> Demux/1
  Demux/3 -> Scope5/2, Multiport Switch/3  "roll angular acceleration"
  Bike Model Parameters1/1 -> Linear Bicycle Model/4(parameters_model)
  Measured Velocity/1 -> Linear Bicycle Model1/3(velocity), Linear Bicycle Model/3(velocity)
  Mux/1 -> Linear Bicycle Model/1(states)
  Roll Angle/1 -> Mux/1
  Steering Angle/1 -> Multiport Switch1/2, Mux/2
  Constant/1 -> Multiport Switch/1
  Multiport Switch/1 -> Multiply1/2
  Demux1/3 -> Scope5/3, Multiport Switch/4  "roll angular acceleration"
  Bike Model Parameters2/1 -> Linear Bicycle Model1/4(parameters_model)
  Delay/1 -> Demux3/1, Sum/2  "x"
  Multiply/1 -> Sum/1
  Constant2/1 -> Multiply/1
  Integrator/1 -> Linear Bicycle Model1/1(states), Demux2/1  "x"
  Demux2/1 -> Mux1/1
  Demux3/1 -> Mux1/2
  Demux2/2 -> Mux2/1
  Demux3/2 -> Mux2/2
  Demux2/3 -> Mux3/1
  Demux3/3 -> Mux3/2
  Mux2/1 -> Scope/2
  Mux1/1 -> Scope6/1, Scope/1
  Mux3/1 -> Scope/3
  Linear Bicycle Model1/1(xdot) -> Multiply/2, Demux1/1, Integrator/1
  State-Space/1 -> Scope3/1
  Delay1/1 -> Scope4/1, discrete/1(states)
  Zero-Order Hold/1 -> Scope2/1, Subsystem/1(In1)
  discrete/1(x_next) -> Delay1/1
  Constant5/1 -> discrete/4(B)
  Constant3/1 -> discrete/3(A)
  Sum/1 -> Delay/1  "x_next"
  Zero-Order Hold1/1 -> discrete/2(input), Scope1/1
  Multiport Switch1/1 -> Steering Angle (temporary output)/1
  Constant1/1 -> Multiport Switch1/1
  Steering Rate/1 -> Zero-Order Hold/1, State-Space/1, Discrete State-Space/1, Zero-Order Hold1/1, Linear Bicycle Model1/2(input), Linear Bicycle Model/2(input)
  Integrator1/1 -> Multiport Switch1/3
  Demux/2 -> Integrator1/1
  Demux1/2 -> Integrator2/1
  Integrator2/1 -> Multiport Switch1/4
  Demux4/1 -> Scope6/2
  Demux5/1 -> Scope6/3
  Discrete State-Space/1 -> Demux4/1
  Subsystem/1(Out1) -> Demux5/1

== system bike_model_2states_smithSteering/Physical Bike/Global Angles and Coordinates Calculator - Position/Measured Bike Angles to Global Angles ==
  Velocity : Inport
  Measured Steering Angle : Inport  Port=2
  " Bike Parameters Model " : Constant  Value=parameters_compFilter
  Integrator : Integrator
  MATLAB Function : MATLAB Function  TreatAsAtomicUnit=on
  To Workspace6 : ToWorkspace  VariableName=PSI  SaveFormat=Timeseries  SampleTime=Ts
  To Workspace7 : ToWorkspace  VariableName=BETA  SaveFormat=Timeseries  SampleTime=Ts
  Psi : Outport
  Beta : Outport  Port=2
  wires:
  MATLAB Function/2(beta) -> Beta/1, To Workspace7/1
  MATLAB Function/1(psi_d) -> Integrator/1
  Integrator/1 -> Psi/1, To Workspace6/1
  " Bike Parameters Model "/1 -> MATLAB Function/2(parameters_model)
  Measured Steering Angle/1 -> MATLAB Function/3(delta)
  Velocity/1 -> MATLAB Function/1(v)

== system bike_model_2states_smithSteering/Physical Bike/Global Angles and Coordinates Calculator - Position/Measured Global Angles to Global Coordinates ==
  Velocity : Inport
  Psi : Inport  Port=2
  Beta : Inport  Port=3
  Constant : Constant  Value=initial_y
  Constant1 : Constant  Value=initial_x
  Integrator1 : Integrator
  Integrator2 : Integrator
  MATLAB Function1 : MATLAB Function  TreatAsAtomicUnit=on
  Mux : Mux  Inputs=2
  Sum : Sum  Inputs=|++
  Sum1 : Sum  Inputs=++|
  "Position (X, Y)" : Outport
  wires:
  MATLAB Function1/2(Ydot) -> Integrator2/1  "Ydot"
  MATLAB Function1/1(Xdot) -> Integrator1/1  "Xdot"
  Psi/1 -> MATLAB Function1/2(psi)
  Beta/1 -> MATLAB Function1/3(beta)
  Velocity/1 -> MATLAB Function1/1(v)
  Integrator2/1 -> Sum/1
  Constant/1 -> Sum/2
  Sum/1 -> Mux/2
  Integrator1/1 -> Sum1/2
  Sum1/1 -> Mux/1
  Constant1/1 -> Sum1/1
  Mux/1 -> "Position (X, Y)"/1

== system bike_model_2states_smithSteering/Complementary filter/Roll Angle Estimation of Accelerometer/Lateral Acceleration Compensator/Low Pass Filter ==
  Roll Rate : Inport
  Delay18 : Delay  DelayLength=1  SampleTime=Ts_IMU
  Gain4 : Gain  Gain=roll_rate_coef
  Gain6 : Gain  Gain=1-roll_rate_coef
  Scope7 : Scope  NumInputPorts=2
  Sum4 : Sum  Inputs=|++
  Filtered Roll Rate : Outport
  wires:
  Gain6/1 -> Sum4/1
  Gain4/1 -> Sum4/2
  Sum4/1 -> Filtered Roll Rate/1, Delay18/1, Scope7/2  "Filtered Roll Rate"
  Delay18/1 -> Gain4/1
  Roll Rate/1 -> Scope7/1, Gain6/1  "Measured Roll Rate"
